simulink model "dianji1fuzzypid"  (R2014b)
settings: Solver=ode45  StartTime=0.0  StopTime=10.0  RelTol=1e-3
libraries: simulink x1, fuzblock x1, powerlib x1
settings Model: Creator=Administrator  LastModifiedBy=Administrator

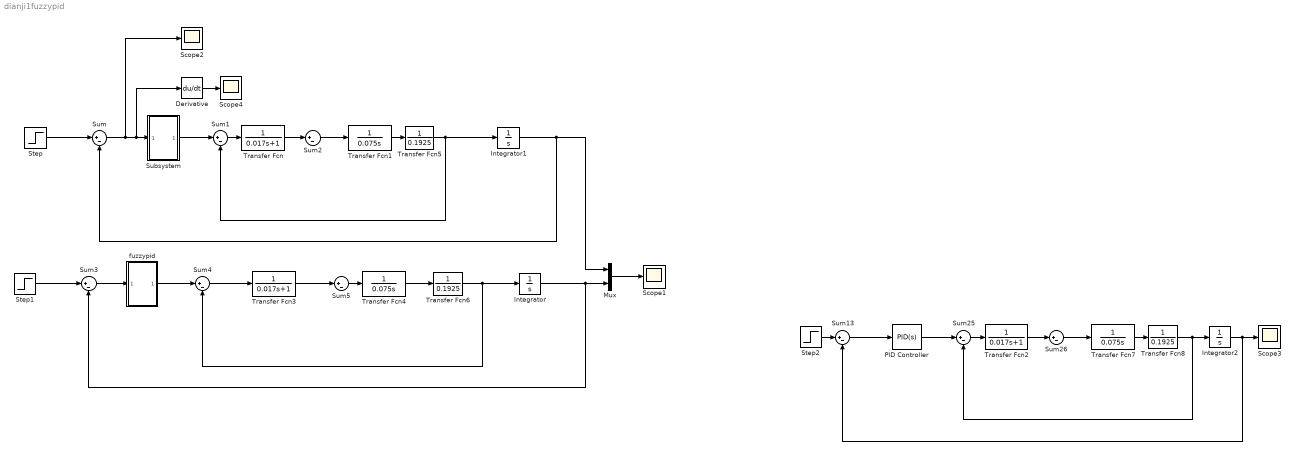
== system dianji1fuzzypid ==
  Derivative : Derivative
  Integrator : Integrator
  Integrator1 : Integrator
  Integrator2 : Integrator
  Mux : Mux  Inputs=2
  PID Controller : simulink/Continuous/PID Controller  Controller=PID  TimeDomain=Continuous-time  SampleTime=-1  IntegratorMethod=Forward Euler  FilterMethod=Forward Euler  Form=Parallel  P=22.0696160979341  I=3.80775639731004  D=-0.39390939873363  N=19.6567757288827  InitialConditionSource=internal  InitialConditionForIntegrator=0  InitialConditionForFilter=0  ExternalReset=none  LimitOutput=off  UpperSaturationLimit=inf  LowerSaturationLimit=-inf  LinearizeAsGain=on  AntiWindupMode=none  Kb=1  TrackingMode=off  Kt=1  PParamMin=[]  PParamMax=[]  IParamMin=[]  IParamMax=[]  DParamMin=[]  DParamMax=[]  NParamMin=[]  NParamMax=[]  KbParamMin=[]  KbParamMax=[]  KtParamMin=[]  KtParamMax=[]  POutMin=[]  POutMax=[]  IOutMin=[]  IOutMax=[]  DOutMin=[]  DOutMax=[]  NOutMin=[]  NOutMax=[]  KbOutMin=[]  KbOutMax=[]  KtOutMin=[]  KtOutMax=[]  IntegratorOutMin=[]  IntegratorOutMax=[]  FilterOutMin=[]  FilterOutMax=[]  SumOutMin=[]  SumOutMax=[]  SumI1OutMin=[]  SumI1OutMax=[]  SumI2OutMin=[]  SumI2OutMax=[]  SumI3OutMin=[]  SumI3OutMax=[]  SumDOutMin=[]  SumDOutMax=[]  SaturationOutMin=[]  SaturationOutMax=[]  IntegratorContinuousStateAttributes=''  IntegratorStateMustResolveToSignalObject=off  IntegratorRTWStateStorageClass=Auto  FilterContinuousStateAttributes=''  FilterStateMustResolveToSignalObject=off  FilterRTWStateStorageClass=Auto  DifferentiatorICPrevScaledInput=0  DifferentiatorOutMin=[]  DifferentiatorOutMax=[]  UseFilter=on
  Scope{1..4} (4 alike) : Scope
      Scope1 settings: YMin=-1.2e-11  YMax=0
      Scope2 settings: YMin=-1.2e-11  YMax=0  SaveName=ScopeData3
      Scope3 settings: YMin=-1.2e-11  YMax=0
      Scope4 settings: YMin=-1.2e-11  YMax=0  SaveName=ScopeData4
  Step : Step  After=50  SampleTime=0
  Step1 : Step  After=50  SampleTime=0
  Step2 : Step  After=50  SampleTime=0
  Subsystem : Subsystem
  Sum{,1..5,13,25..26} (9 alike) : Sum  Inputs=|+-
  Transfer Fcn : TransferFcn  Denominator=[0.017 1]
  Transfer Fcn1 : TransferFcn  Denominator=[0.075 0]
  Transfer Fcn2 : TransferFcn  Denominator=[0.017 1]
  Transfer Fcn3 : TransferFcn  Denominator=[0.017 1]
  Transfer Fcn4 : TransferFcn  Denominator=[0.075 0]
  Transfer Fcn5 : TransferFcn  Denominator=[0.1925]
  Transfer Fcn6 : TransferFcn  Denominator=[0.1925]
  Transfer Fcn7 : TransferFcn  Denominator=[0.075 0]
  Transfer Fcn8 : TransferFcn  Denominator=[0.1925]
  fuzzypid : Subsystem
  wires:
  Transfer Fcn1/1 -> Transfer Fcn5/1
  Step/1 -> Sum/1
  Sum1/1 -> Transfer Fcn/1
  Integrator1/1 -> Sum/2, Mux/1
  Transfer Fcn/1 -> Sum2/1
  Sum2/1 -> Transfer Fcn1/1
  Transfer Fcn4/1 -> Transfer Fcn6/1
  Step1/1 -> Sum3/1
  Sum4/1 -> Transfer Fcn3/1
  Transfer Fcn3/1 -> Sum5/1
  Sum5/1 -> Transfer Fcn4/1
  Mux/1 -> Scope1/1
  Integrator/1 -> Mux/2, Sum3/2
  Sum3/1 -> fuzzypid/1(In1)
  fuzzypid/1(Out1) -> Sum4/1
  Subsystem/1(Out1) -> Sum1/1
  Transfer Fcn6/1 -> Integrator/1, Sum4/2
  Transfer Fcn5/1 -> Integrator1/1, Sum1/2
  Transfer Fcn7/1 -> Transfer Fcn8/1
  Step2/1 -> Sum13/1
  Sum25/1 -> Transfer Fcn2/1
  Transfer Fcn2/1 -> Sum26/1
  Sum26/1 -> Transfer Fcn7/1
  Sum13/1 -> PID Controller/1
  PID Controller/1 -> Sum25/1
  Transfer Fcn8/1 -> Integrator2/1, Sum25/2
  Integrator2/1 -> Scope3/1, Sum13/2
  Sum/1 -> Scope2/1, Derivative/1, Subsystem/1(In1)
  Derivative/1 -> Scope4/1

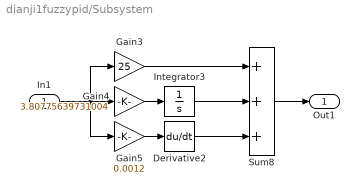
== system dianji1fuzzypid/Subsystem ==
  In1 : Inport
  Derivative2 : Derivative
  Gain3 : Gain  Gain=25
  Gain4 : Gain  Gain=3.80775639731004
  Gain5 : Gain  Gain=0.0012
  Integrator3 : Integrator
  Sum8 : Sum  Inputs=+++
  Out1 : Outport
  wires:
  Gain4/1 -> Integrator3/1
  Gain3/1 -> Sum8/1
  Derivative2/1 -> Sum8/3
  Gain5/1 -> Derivative2/1
  Sum8/1 -> Out1/1
  In1/1 -> Gain5/1, Gain4/1, Gain3/1
  Integrator3/1 -> Sum8/2

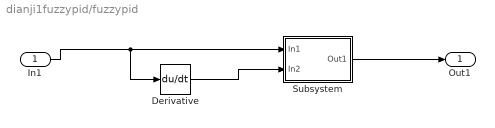
== system dianji1fuzzypid/fuzzypid ==
  In1 : Inport
  Derivative : Derivative
  Subsystem : Subsystem
  Out1 : Outport
  wires:
  Subsystem/1(Out1) -> Out1/1
  Derivative/1 -> Subsystem/2(In2)
  In1/1 -> Derivative/1, Subsystem/1(In1)

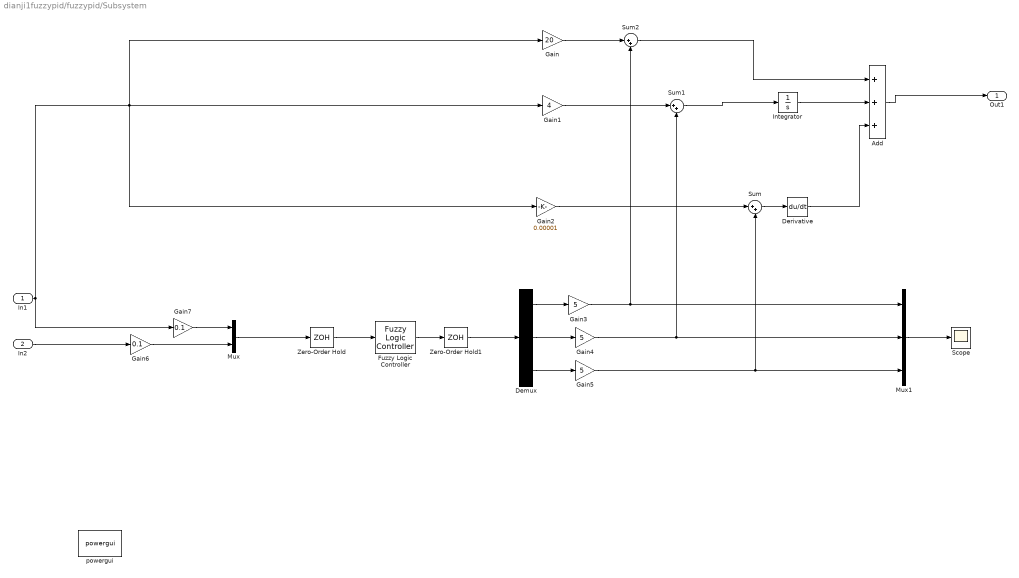
== system dianji1fuzzypid/fuzzypid/Subsystem ==
  In1 : Inport
  In2 : Inport  Port=2
  Add : Sum  Inputs=+++
  Demux : Demux  Outputs=3
  Derivative : Derivative
  Fuzzy Logic Controller : fuzblock/Fuzzy Logic  Controller  fis=fuzzy_1
  Gain : Gain  Gain=20
  Gain1 : Gain  Gain=4
  Gain2 : Gain  Gain=0.00001
  Gain3 : Gain  Gain=5
  Gain4 : Gain  Gain=5
  Gain5 : Gain  Gain=5
  Gain6 : Gain  Gain=0.1
  Gain7 : Gain  Gain=0.1
  Integrator : Integrator
  Mux : Mux  Inputs=2
  Mux1 : Mux  Inputs=3
  Scope : Scope
      settings: SaveName=ScopeData2
  Sum : Sum  Inputs=|++
  Sum1 : Sum  Inputs=|++
  Sum2 : Sum  Inputs=|++
  Zero-Order Hold : ZeroOrderHold  SampleTime=0.01
  Zero-Order Hold1 : ZeroOrderHold  SampleTime=0.01
  powergui : powerlib/powergui  Priority=1  SimulationMode=Continuous  SolverType=Tustin/Backward Euler (TBE)  SampleTime=50e-6  frequency=60  SPID=off  DisableSnubberDevices=off  DisableRonSwitches=off  DisableVfSwitches=off  SwTol=0  DisplayEquations=off  Interpol=off  methode=off  Ts=100  frequencyindice=60  Pbase=100e6  ErrMax=1e-4  Iterations=50  UnitsV=kV  UnitsW=MW  FunctionMessages=off  echomessages=off  HookPort=off  EnableUseOfTLC=off  x0status=blocks  RestoreLinks=warning  ResistiveCurrentMeasurement=off  Frange=[0:2:500]  Ylog=off  Xlog=on  ShowGrid=off  save=off  variable=ZData  structure=0  ZoomFFT=off  StartTime=0.0  cycles=1  DisplayStyle=1  fundamental=60  FreqAxis=off  MaxFrequency=1000  frequencyindicesteady=1  RmsSteady=1  display=off
  Out1 : Outport
  wires:
  In1/1 -> Gain/1, Gain2/1, Gain1/1, Gain7/1
  Derivative/1 -> Add/3
  Integrator/1 -> Add/2
  Add/1 -> Out1/1
  In2/1 -> Gain6/1
  Gain/1 -> Sum2/1
  Sum2/1 -> Add/1
  Gain1/1 -> Sum1/1
  Sum1/1 -> Integrator/1
  Gain2/1 -> Sum/1
  Sum/1 -> Derivative/1
  Mux/1 -> Zero-Order Hold/1
  Fuzzy Logic Controller/1 -> Zero-Order Hold1/1
  Zero-Order Hold/1 -> Fuzzy Logic Controller/1
  Zero-Order Hold1/1 -> Demux/1
  Demux/1 -> Gain3/1
  Demux/2 -> Gain4/1
  Demux/3 -> Gain5/1
  Mux1/1 -> Scope/1
  Gain3/1 -> Mux1/1, Sum2/2
  Gain4/1 -> Mux1/2, Sum1/2
  Gain5/1 -> Mux1/3, Sum/2
  Gain7/1 -> Mux/1
  Gain6/1 -> Mux/2
